simulink subsystem "Sonars"  (R2022b)
settings: Solver=VariableStepAuto  StartTime=0.0  StopTime=10.0  RelTol=1e-3
libraries: arduinolib x2
settings Model: Creator=dar.io  LastModifiedBy=dar.io

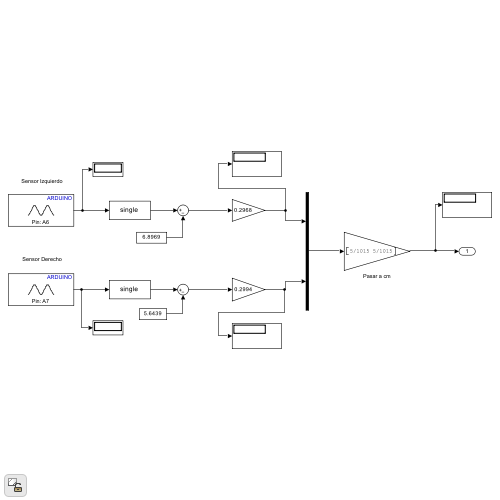
[thumbnail: Simulink's stored preview of the top-level diagram]
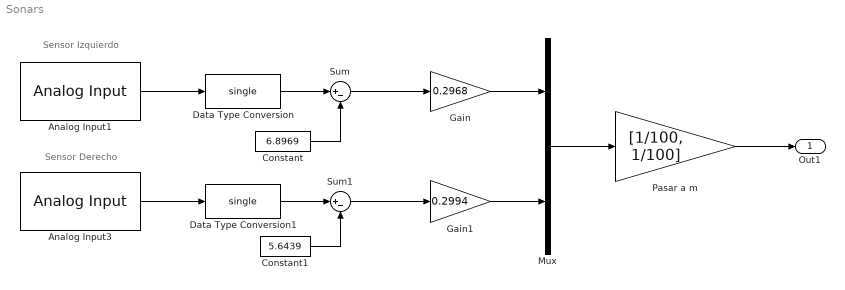
== system Sonars ==
  note: Sensor Izquierdo
  note: Sensor Derecho
  Analog Input1 : arduinolib/Analog Input  pinNumber=6  ReadResultsOnly=off  ConversionTriggerSource=Software  ExternalTriggerType=uint32( 0 )  OutputDataType=uint16  EnableConversionCompleteNotify=off  EnableOuputStatus=off  SampleTime=-1  blockPlatform=arduino
  Analog Input3 : arduinolib/Analog Input  pinNumber=7  ReadResultsOnly=off  ConversionTriggerSource=Software  ExternalTriggerType=uint32( 0 )  OutputDataType=uint16  EnableConversionCompleteNotify=off  EnableOuputStatus=off  SampleTime=-1  blockPlatform=arduino
  Constant : Constant  Value=6.8969
  Constant1 : Constant  Value=5.6439
  Data Type Conversion : DataTypeConversion  OutDataTypeStr=single  SaturateOnIntegerOverflow=off  RndMeth=Floor
  Data Type Conversion1 : DataTypeConversion  OutDataTypeStr=single  SaturateOnIntegerOverflow=off  RndMeth=Floor
  Gain : Gain  Gain=0.2968
  Gain1 : Gain  Gain=0.2994
  Mux : Mux  Inputs=2
  Pasar a m : Gain  Gain=[1/100, 1/100]
  Sum : Sum  Inputs=|+-
  Sum1 : Sum  Inputs=|+-
  Out1 : Outport
  wires:
  Constant/1 -> Sum/2
  Data Type Conversion/1 -> Sum/1
  Gain1/1 -> Mux/2
  Sum/1 -> Gain/1
  Sum1/1 -> Gain1/1
  Analog Input3/1 -> Data Type Conversion1/1
  Mux/1 -> Pasar a m/1
  Data Type Conversion1/1 -> Sum1/1
  Constant1/1 -> Sum1/2
  Pasar a m/1 -> Out1/1
  Analog Input1/1 -> Data Type Conversion/1
  Gain/1 -> Mux/1
